simulink model "trajectory_simulation"  (R2018b)
settings: Solver=ode4  StartTime=0.0  StopTime=25  FixedStep=1e-4  RelTol=1e-3
undefined symbols (not defined in the file or in its folder): xi_0
settings Model: Creator=edoz9  LastModifiedBy=Stefano
settings DataIOCC: SaveOutput=off  SignalLogging=off  DSMLogging=off  SaveTime=off
settings OptimizationCC: DefaultParameterBehavior=Inlined  UseDivisionForNetSlopeComputation=on  UseFloatMulNetSlope=on  InlineInvariantSignals=on  PassReuseOutputArgsAs=Individual arguments  ZeroExternalMemoryAtStartup=off  ZeroInternalMemoryAtStartup=off  NoFixptDivByZeroProtection=on  EfficientFloat2IntCast=on  LifeSpan=1  OptimizeBlockOrder=speed  DifferentSizesBufferReuse=on
settings DebuggingCC: ParameterTunabilityLossMsg=error  UnderSpecifiedDimensionMsg=warning
settings HardwareCC: ProdLongLongMode=on
settings SFSimCC: MATLABDynamicMemAlloc=off
settings RTWCC: SystemTargetFile=ert.tlc  GenCodeOnly=on  TemplateMakefile=ert_default_tmf  GenerateReport=on  IncludeHyperlinkInReport=on  LaunchReport=on  GenerateTraceInfo=on  GenerateTraceReport=on  GenerateTraceReportSl=on  GenerateTraceReportSf=on  GenerateTraceReportEml=on  GenerateCodeMetricsReport=on
settings CodeAppCC: ForceParamTrailComments=on  IgnoreCustomStorageClasses=off  OperatorAnnotations=on  SimulinkDataObjDesc=on  SFDataObjDesc=on  CustomSymbolStrGlobalVar=rt$N$M  CustomSymbolStrType=$N$M  CustomSymbolStrFcn=$N$M$F  CustomSymbolStrMacro=$N$M  InsertBlockDesc=on
settings ERTTargetCC: TargetLangStandard=C99 (ISO)  GenerateSampleERTMain=on  IncludeMdlTerminateFcn=off  CombineSignalStateStructs=on  SupportAbsoluteTime=off  SupportComplex=off  SupportContinuousTime=on  SupportNonInlinedSFcns=on  InlinedParameterPlacement=NonHierarchical  ERTCustomFileTemplate=example_file_process.tlc  ERTFilePackagingFormat=CompactWithDataFile

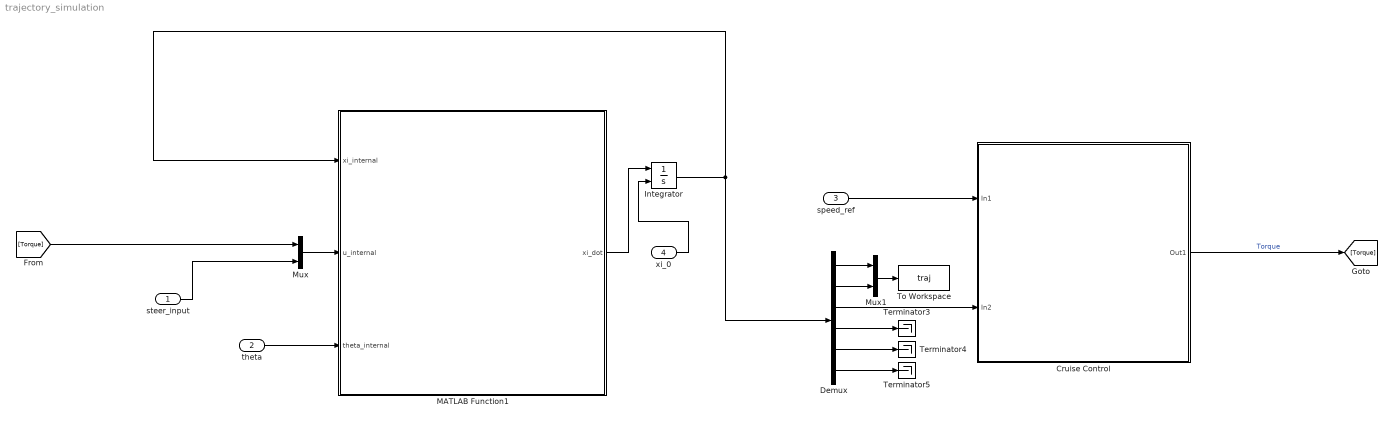
== system trajectory_simulation ==
  steer_input : Inport  OutDataTypeStr=double  PortDimensions=1
  theta : Inport  Port=2  OutDataTypeStr=double  PortDimensions=13
  speed_ref : Inport  Port=3  OutDataTypeStr=double  PortDimensions=1
  xi_0 : Inport  Port=4  OutDataTypeStr=double  PortDimensions=6
  Cruise Control : Subsystem
  Demux : Demux  Outputs=6
  Integrator : Integrator  InitialConditionSource=external  InitialCondition=xi_0
  MATLAB Function1 : MATLAB Function  TreatAsAtomicUnit=on
  Mux : Mux  Inputs=2
  Mux1 : Mux  Inputs=2
  Terminator3 : Terminator
  Terminator4 : Terminator
  Terminator5 : Terminator
  To Workspace : ToWorkspace  VariableName=traj  SaveFormat=Structure With Time  SampleTime=-1
  wires:
  steer_input/1 -> Mux/2
  Cruise Control/1(Out1) -> [Torque]  "Torque"
  [Torque] -> Mux/1
  speed_ref/1 -> Cruise Control/1(In1)
  Demux/3 -> Cruise Control/2(In2)
  Demux/1 -> Mux1/1
  Demux/2 -> Mux1/2
  Demux/4 -> Terminator3/1
  Demux/5 -> Terminator4/1
  Demux/6 -> Terminator5/1
  Integrator/1 -> Demux/1, MATLAB Function1/1(xi_internal)
  MATLAB Function1/1(xi_dot) -> Integrator/1
  theta/1 -> MATLAB Function1/3(theta_internal)
  Mux/1 -> MATLAB Function1/2(u_internal)
  xi_0/1 -> Integrator/2
  Mux1/1 -> To Workspace/1

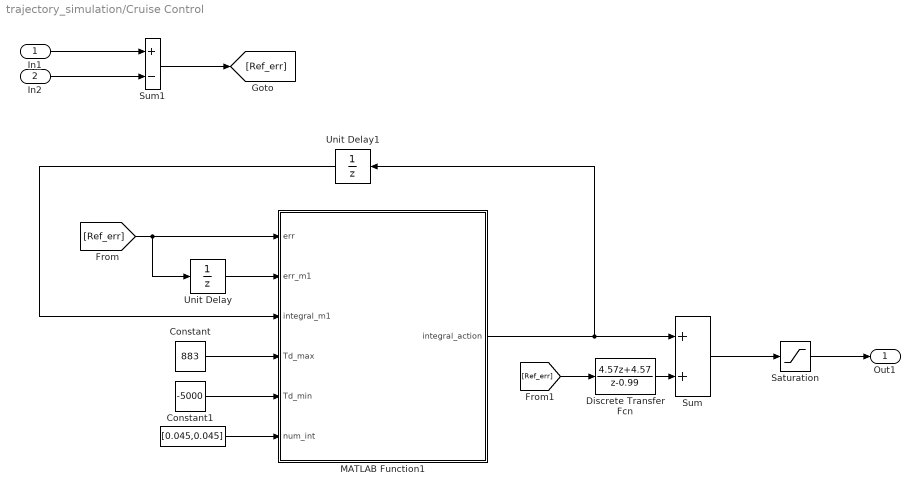
== system trajectory_simulation/Cruise Control ==
  In1 : Inport
  In2 : Inport  Port=2
  "  " : Constant  Value=[0.045,0.045]
  Constant : Constant  Value=883
  Constant1 : Constant  Value=-5000
  Discrete Transfer Fcn : DiscreteTransferFcn  Numerator=[ 4.57,4.57 ]  Denominator=[ 1,-0.99 ]
  MATLAB Function1 : MATLAB Function  TreatAsAtomicUnit=on
  Saturation : Saturate  UpperLimit=883  LowerLimit=-5000
  Sum : Sum
  Sum1 : Sum  Inputs=+-
  Unit Delay : UnitDelay  SampleTime=-1
  Unit Delay1 : UnitDelay  SampleTime=-1
  Out1 : Outport
  wires:
  Constant1/1 -> MATLAB Function1/5(Td_min)
  Unit Delay/1 -> MATLAB Function1/2(err_m1)
  [Ref_err] -> Unit Delay/1, MATLAB Function1/1(err)
  Constant/1 -> MATLAB Function1/4(Td_max)
  MATLAB Function1/1(integral_action) -> Sum/1, Unit Delay1/1
  Discrete Transfer Fcn/1 -> Sum/2
  Sum/1 -> Saturation/1
  In1/1 -> Sum1/1
  In2/1 -> Sum1/2
  Sum1/1 -> [Ref_err]
  [Ref_err] -> Discrete Transfer Fcn/1
  Saturation/1 -> Out1/1
  "  "/1 -> MATLAB Function1/6(num_int)
  Unit Delay1/1 -> MATLAB Function1/3(integral_m1)

== matlab function trajectory_simulation/Cruise Control/MATLAB Function1 ==
  data: err input; integral_action output; err_m1 input; integral_m1 input; Td_max input; Td_min input; num_int input
function integral_action = integrator_anti_wu(err, err_m1, integral_m1, Td_max, Td_min, num_int)

integral_action = min(Td_max, max(Td_min, integral_m1+num_int'*[err;err_m1]));

== matlab function trajectory_simulation/MATLAB Function1 ==
  data: xi_internal input; u_internal input; xi_dot output; theta_internal input
function xi_dot = vehicle(xi_internal, u_internal, theta_internal)
% simulation, time has to be the fist input

%% Read states
X = xi_internal(1,1);
Y = xi_internal(2,1);
Ux = xi_internal(3,1);
beta = xi_internal(4,1);
psi = xi_internal(5,1);
r = xi_internal(6,1);

%% Read Inputs

Td_internal = u_internal(1,1);
delta_internal = u_internal(2,1);

%% Read Parameters

m = theta_internal(1,1);
Jz = theta_internal(2,1);
a = theta_internal(3,1);
b = theta_internal(4,1);
Cf = theta_internal(5,1);
Cr = theta_internal(6,1);
rw = theta_internal(7,1);
mu = theta_internal(8,1);
Af = theta_internal(9,1);
Al = theta_internal(10,1);
Cx = theta_internal(11,1);
Rr = theta_internal(12,1);
rho = theta_internal(13,1);
g = 9.81;

%% Equations

Uy = tan(beta)*Ux;
alfa_f = atan2((Uy + a*r),Ux) - delta_internal;
alfa_r = atan2((Uy - b*r),Ux);

F_z_f = m * g * b / (a+b);
F_z_r = m * g * a / (a+b);

z_f = tan(alfa_f);
z_r = tan(alfa_r);

elem1 = mu*F_z_f;
elem21 = - mu*F_z_f;
elem22 = - Cf*z_f + (Cf^2*abs(z_f)*z_f)/(3*mu*F_z_f) - (Cf^3*z_f^3)/(27*mu^2*F_z_f^2);
elem2 = max(elem21,elem22);
F_y_f = min(elem1, elem2);

elem1 = mu*F_z_r;
elem21 = - mu*F_z_r;
elem22 = - Cr*z_r + (Cr^2*abs(z_r)*z_r)/(3*mu*F_z_r) - (Cr^3*z_r^3)/(27*mu^2*F_z_r^2);
elem2 = max(elem21,elem22);
F_y_r = min(elem1,elem2);

F_x = Td_internal/rw;

F_r = Rr*Ux;
F_x_d = 0.5*rho*Af*Cx*Ux^2;

%% Output
xi_dot = zeros(6,1);
xi_dot(1,1) = Ux*cos(psi) - Uy*sin(psi);
xi_dot(2,1) = Ux*sin(psi)+ Uy*cos(psi);
xi_dot(3,1) = 1/m * ((F_x - F_y_f*sin(delta_internal))-F_r-F_x_d);
xi_dot(4,1) = 1/(m*Ux) * (F_y_f*cos(delta_internal)+F_y_r) - r;
xi_dot(5,1) = r;
xi_dot(6,1) = 1/Jz * (a*F_y_f*cos(delta_internal) - b* F_y_r);
% Forces = zeros(3,1);
% Forces(1,1) = F_y_f;
% Forces(2,1) = F_y_r;
% Forces(3,1) = F_x;

end
